simulink model "Par_RLC_Sys"  (R2015a)
settings: Solver=ode23  StartTime=0.0  StopTime=10  RelTol=1e-3
settings Model: Creator=Kunal  LastModifiedBy=Kunal
settings SolverCC: AutoInsertRateTranBlk=on

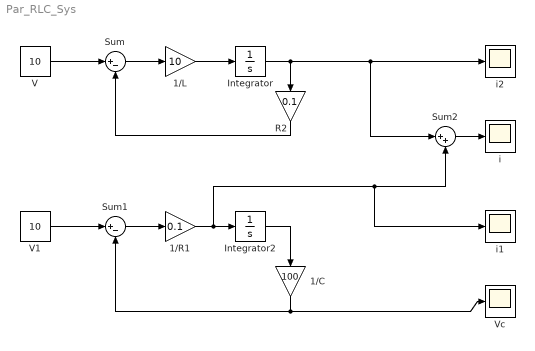
== system Par_RLC_Sys ==
  1/C : Gain  Gain=100
  1/L : Gain  Gain=10
  1/R1 : Gain  Gain=0.1
  Integrator : Integrator
  Integrator2 : Integrator
  R2 : Gain  Gain=0.1
  Sum : Sum  Inputs=|+-
  Sum1 : Sum  Inputs=|+-
  Sum2 : Sum  Inputs=|++
  V : Constant  Value=10
  V1 : Constant  Value=10
  Vc : Scope
  i : Scope
      settings: YMax=110
  i1 : Scope
      settings: SaveName=ScopeData2
  i2 : Scope
      settings: SaveName=ScopeData3
  wires:
  Integrator/1 -> i2/1, Sum2/1, R2/1
  R2/1 -> Sum/2
  Sum/1 -> 1/L/1
  V/1 -> Sum/1
  1/L/1 -> Integrator/1
  Integrator2/1 -> 1/C/1
  1/C/1 -> Vc/1, Sum1/2
  Sum1/1 -> 1/R1/1
  V1/1 -> Sum1/1
  1/R1/1 -> i1/1, Sum2/2, Integrator2/1
  Sum2/1 -> i/1
